simulink model "Longitudinal_Test"  (R2023b)
settings: Solver=VariableStepAuto  StartTime=0.0  StopTime=10.0  RelTol=1e-3
settings Model: Creator=Ahmed Raamadan  LastModifiedBy=Ahmed Raamadan

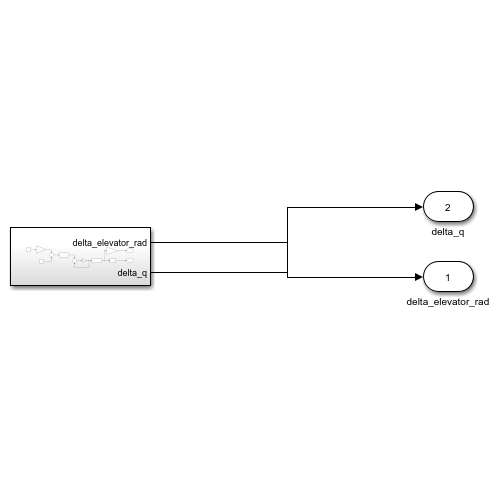
[thumbnail: Simulink's stored preview of the top-level diagram]
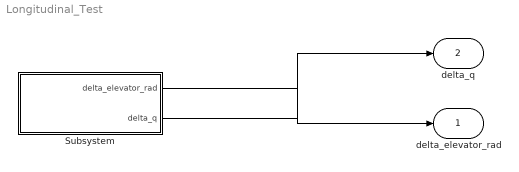
== system Longitudinal_Test ==
  Subsystem : Subsystem
  delta_elevator_rad : Outport
  delta_q : Outport  Port=2
  wires:
  Subsystem/1(delta_elevator_rad) -> delta_elevator_rad/1
  Subsystem/2(delta_q) -> delta_q/1

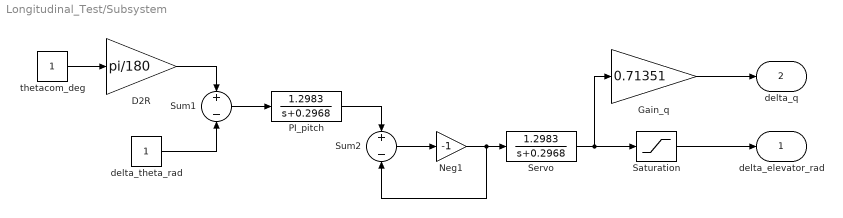
== system Longitudinal_Test/Subsystem ==
  D2R : Gain  Gain=pi/180
  Gain_q : Gain  Gain=0.71351
  Neg1 : Gain  Gain=-1
  PI_pitch : TransferFcn  Numerator=[1.2983]  Denominator=[1 0.2968]
  Saturation : Saturate  UpperLimit=inf  LowerLimit=-inf
  Servo : TransferFcn  Numerator=1.2983  Denominator=[1 0.2968]
  Sum1 : Sum  Inputs=+-
  Sum2 : Sum  Inputs=+-
  delta_theta_rad : Constant
  thetacom_deg : Constant
  delta_elevator_rad : Outport
  delta_q : Outport  Port=2
  wires:
  delta_theta_rad/1 -> Sum1/2
  thetacom_deg/1 -> D2R/1
  Saturation/1 -> delta_elevator_rad/1
  Neg1/1 -> Sum2/2, Servo/1
  Servo/1 -> Saturation/1, Gain_q/1
  Sum1/1 -> PI_pitch/1
  PI_pitch/1 -> Sum2/1
  Sum2/1 -> Neg1/1
  D2R/1 -> Sum1/1
  Gain_q/1 -> delta_q/1
